simulink library "RTMDblocks"  (Simulink 7.0)
undefined symbols (not defined in the file or in its folder): node, sample
libraries: xpcsystranlib x3, xpclib x1
settings Model: Creator=Tommy  LastModifiedBy=Tommy

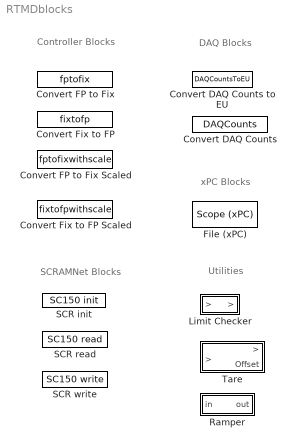
== system RTMDblocks ==
  note: Controller Blocks
  note: DAQ Blocks
  note: SCRAMNet Blocks
  note: xPC Blocks
  note: Utilities
  Convert DAQ Counts : S-Function  FunctionName=DAQCounts  SFunctionModules=DAQCounts_wrapper
      mask Type: DAQCounts
      mask Description: Convert uint32 Raw Counts to signed int32 Counts
      mask Display:
      | port_label('input',1,'Counts')
      | port_label('output',1,'Counts')
  Convert DAQ Counts to EU : S-Function  FunctionName=DAQCountsToEU  Parameters=gain,Vslope,Voffset,EUslope,EUoffset  SFunctionModules=DAQCountsToEU_wrapper  mask(DAQCountsToEU){gain=0, Vslope=0, Voffset=0, EUslope=0, EUoffset=0}
      mask help: Convert DAQ Counts to Engineering Units
      mask Display:
      | port_label('input',1,'Counts')
      | port_label('output',1,'EU')
  Convert FP to Fix : S-Function  FunctionName=fptofix  SFunctionModules=fptofix_wrapper
      mask Type: FPtoFix
      mask Description: Convert Floating Point value to uint32 Fixed Point
      mask Display:
      | port_label('input',1,'Float')
      | port_label('output',1,'Fixed')
  Convert FP to Fix Scaled : S-Function  FunctionName=fptofixwithscale  Parameters=scale  SFunctionModules=fptofixwithscale_wrapper  mask(FPtoFixScaled){scale=1}
      mask help: Convert Floating Point value to uint32 Fixed Point and scale to normalized value.
      mask Display:
      | port_label('input',1,'Float')
      | port_label('output',1,'Fixed')
      | fprintf('1/%d',scale);
  Convert Fix to FP : S-Function  FunctionName=fixtofp  SFunctionModules=fixtofp_wrapper
      mask Type: FixtoFP
      mask Description: Convert uint32 Fixed Point to Floating Point
      mask Display:
      | port_label('input',1,'Fixed')
      | port_label('output',1,'Float')
  Convert Fix to FP Scaled : S-Function  FunctionName=fixtofpwithscale  Parameters=scale  SFunctionModules=fixtofpwithscale_wrapper  mask(FixtoFPScaled){scale=1}
      mask help: Convert uint32 Fixed Point to Floating Point and scale
      mask Display:
      | port_label('input',1,'Fixed')
      | port_label('output',1,'Float')
      | fprintf('%d',scale);
  "File (xPC) " : xpclib/Misc./Scope (xPC)   SystemSampleTime=-1  scopeno=1  scopetype=File  autostart=on  viewmode=Graphical redraw  formatstr='%15.6f'  grid=on  ylimits=[0,0]  nosamples=250  noprepostsamples=0  interleave=1  triggermode=FreeRun  triggersignal=1  triggerlevel=0.0  triggerslope=Either  triggerscope=1  triggersample=0  filename=data.dat  mode=Lazy  writesize=512  autorestart=on
  Limit Checker : Subsystem  mask(Limit Checker){upperlimit=1, lowerlimit=-1}
      mask help: Checks if the input signal is within the limits specified and passes it through if true. Otherwise, it will stop the simulation.
  Ramper : Subsystem  mask{ramps=1, samplerate=1/1024, u_old=[0]}
      mask prompts: ramps "Total ramp steps"; samplerate "Sample rate"; u_old "Dimensions"
      mask help:
      | Signal ramper
      |
      | Sample rate should be the sample rate of the system
      | The source signal sample rate should be the sample rate * total ramp steps
      | Set Dimension variable to an empty array of required size, ie. [0;0;0] for 3 dimensions
      mask Display:
      | fprintf('%d',ramps)
      | port_label('input',1,'>')
      | port_label('output',1,'>')
  "SCR init " : xpcsystranlib/Shared Memory/SC150 init   node=[node]  pci=-1
  "SCR read " : xpcsystranlib/Shared Memory/SC150 read   partition=[]  errorport=off  ts=sample  pci=-1
  "SCR write " : xpcsystranlib/Shared Memory/SC150 write   partition=[]  errorport=off  ts=sample  pci=-1
  Tare : Subsystem
      mask Type: Tare Signal
      mask Description:
      | Takes the initial value of a signal and subtracts the signal by that value to produce a tared output.
      | 
      | The Offset output is the constant offset value used to subtract from the signal.

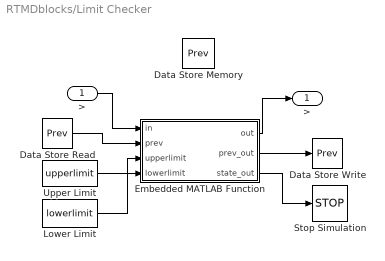
== system RTMDblocks/Limit Checker ==
  > : Inport  OutDataType=sfix(16)  OutScaling=2^0
  Data Store Memory : DataStoreMemory  DataStoreName=Prev  OutDataType=sfix(16)  OutScaling=2^0
  Data Store Read : DataStoreRead  DataStoreName=Prev  SampleTime=sample
  Data Store Write : DataStoreWrite  DataStoreName=Prev  SampleTime=-1
  Embedded MATLAB Function : Stateflow chart
  Lower Limit : Constant  Value=lowerlimit  OutDataType=sfix(16)  OutScaling=2^0
  Stop Simulation : Stop
  Upper Limit : Constant  Value=upperlimit  OutDataType=sfix(16)  OutScaling=2^0
  " >" : Outport  OutDataType=sfix(16)  OutScaling=2^0
  wires:
  Embedded MATLAB Function/2(prev_out) -> Data Store Write/1
  Data Store Read/1 -> Embedded MATLAB Function/2(prev)
  Upper Limit/1 -> Embedded MATLAB Function/3(upperlimit)
  Lower Limit/1 -> Embedded MATLAB Function/4(lowerlimit)
  >/1 -> Embedded MATLAB Function/1(in)
  Embedded MATLAB Function/1(out) -> " >"/1
  Embedded MATLAB Function/3(state_out) -> Stop Simulation/1

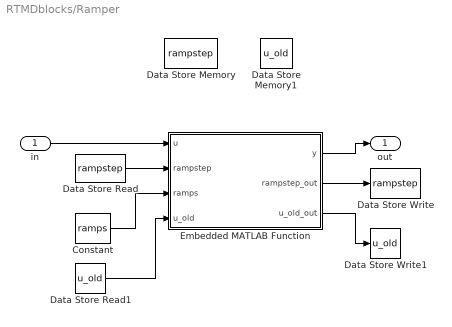
== system RTMDblocks/Ramper ==
  in : Inport  OutDataType=sfix(16)  OutScaling=2^0
  Constant : Constant  Value=ramps  OutDataType=sfix(16)  OutScaling=2^0  SampleTime=samplerate
  Data Store Memory : DataStoreMemory  DataStoreName=rampstep  InitialValue=1  OutDataType=sfix(16)  OutScaling=2^0
  Data Store Memory1 : DataStoreMemory  DataStoreName=u_old  InitialValue=u_old  OutDataType=sfix(16)  OutScaling=2^0
  Data Store Read : DataStoreRead  DataStoreName=rampstep  SampleTime=samplerate
  Data Store Read1 : DataStoreRead  DataStoreName=u_old  SampleTime=samplerate
  Data Store Write : DataStoreWrite  DataStoreName=rampstep  SampleTime=samplerate
  Data Store Write1 : DataStoreWrite  DataStoreName=u_old  SampleTime=samplerate
  Embedded MATLAB Function : Stateflow chart
  out : Outport  OutDataType=sfix(16)  OutScaling=2^0
  wires:
  in/1 -> Embedded MATLAB Function/1(u)
  Data Store Read/1 -> Embedded MATLAB Function/2(rampstep)
  Constant/1 -> Embedded MATLAB Function/3(ramps)
  Data Store Read1/1 -> Embedded MATLAB Function/4(u_old)
  Embedded MATLAB Function/2(rampstep_out) -> Data Store Write/1
  Embedded MATLAB Function/3(u_old_out) -> Data Store Write1/1
  Embedded MATLAB Function/1(y) -> out/1

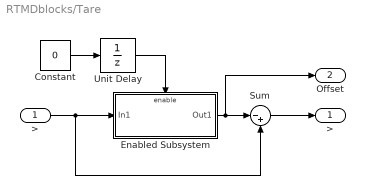
== system RTMDblocks/Tare ==
  > : Inport  OutDataType=sfix(16)  OutScaling=2^0
  Constant : Constant  Value=0  OutDataType=sfix(16)  OutScaling=2^0
  Enabled Subsystem : Subsystem  TreatAsAtomicUnit=on
  Sum : Sum  Inputs=|-+  OutDataType=sfix(16)  OutScaling=2^0
  Unit Delay : UnitDelay  X0=1  SampleTime=-1
  " >" : Outport  OutDataType=sfix(16)  OutScaling=2^0
  Offset : Outport  Port=2  OutDataType=sfix(16)  OutScaling=2^0
  wires:
  >/1 -> Sum/2, Enabled Subsystem/1(In1)
  Enabled Subsystem/1(Out1) -> Offset/1, Sum/1
  Sum/1 -> " >"/1
  Unit Delay/1 -> Enabled Subsystem/Enable
  Constant/1 -> Unit Delay/1

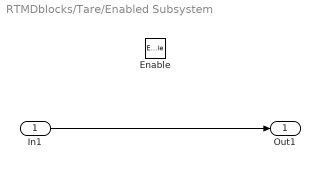
== system RTMDblocks/Tare/Enabled Subsystem ==
  In1 : Inport  OutDataType=sfix(16)  OutScaling=2^0
  Enable : EnablePort
  Out1 : Outport  OutDataType=sfix(16)  OutScaling=2^0
  wires:
  In1/1 -> Out1/1

== matlab function Limit Checker/Embedded MATLAB Function ==
  data: in input inherited; prev input inherited; out output inherited; prev_out output inherited; state_out output inherited; upperlimit input inherited; lowerlimit input inherited
function [out,prev_out,state_out] = fcn(in,prev,upperlimit,lowerlimit)

if ((in < upperlimit) && (in > lowerlimit))
    % ok
    out = in;
    prev_out = in;
    state_out = 0;
else
    % limit hit
    out = prev;
    prev_out = out;
    state_out = 1;
end

== matlab function Ramper/Embedded MATLAB Function ==
  data: u input inherited; y output inherited; rampstep input inherited; ramps input inherited; u_old input inherited; rampstep_out output inherited; u_old_out output inherited
function [y,rampstep_out,u_old_out] = fcn(u,rampstep,ramps,u_old)

%% Ramp
y = (u - u_old)/ramps * rampstep + u_old;    
    
%% Reset ramper
if (rampstep == ramps)
    rampstep_out = 1;
    u_old_out = u; %save this displacement for the base of the next ramped command
else
    rampstep_out = rampstep + 1;
    u_old_out = u_old;
end
